simulink model "part2"  (R2018b)
settings: Solver=VariableStepAuto  StartTime=0.0  StopTime=35  FixedStep=0.01  MaxStep=0.01  RelTol=1e-3
undefined symbols (not defined in the file or in its folder): D, DiscIntNeverNeededParam
libraries: simulink x8, Solver_SF x1, dsparch4 x1
(part 2 of 2)

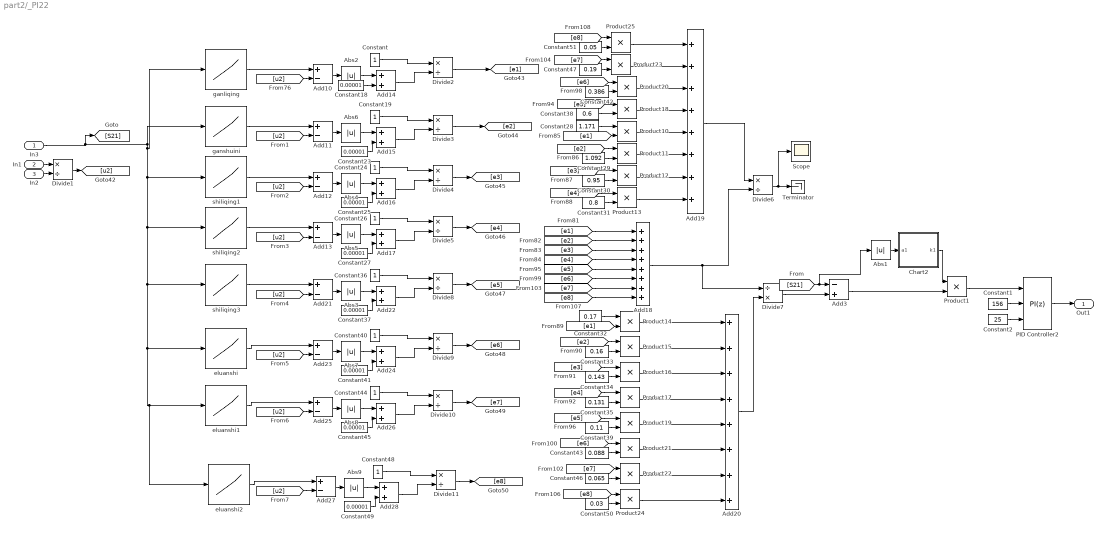
== system part2/_PI22 ==
  In3 : Inport
  In1 : Inport  Port=2
  In2 : Inport  Port=3
  Abs{1..9} (9 alike) : Abs
  Add{10..13,21,23,25,27} (8 alike) : Sum  Inputs=+-
  Add{14..17,22,24,26,28} (8 alike) : Sum
  Add18 : Sum  Inputs=++++++++
  Add19 : Sum  Inputs=++++++++
  Add20 : Sum  Inputs=++++++++
  Add3 : Sum  Inputs=-+
  Chart2 : Stateflow chart  TreatAsAtomicUnit=on
  Constant{,19,24,26,36,40,44,48} (8 alike) : Constant
  Constant1 : Constant  Value=156
  Constant{18,23,25,27,37,41,45,49} (8 alike) : Constant  Value=0.00001
  Constant2 : Constant  Value=25
  Constant28 : Constant  Value=1.171
  Constant29 : Constant  Value=1.092
  Constant30 : Constant  Value=0.95
  Constant31 : Constant  Value=0.8
  Constant32 : Constant  Value=0.17
  Constant33 : Constant  Value=0.16
  Constant34 : Constant  Value=0.143
  Constant35 : Constant  Value=0.131
  Constant38 : Constant  Value=0.6
  Constant39 : Constant  Value=0.11
  Constant42 : Constant  Value=0.386
  Constant43 : Constant  Value=0.088
  Constant46 : Constant  Value=0.065
  Constant47 : Constant  Value=0.19
  Constant50 : Constant  Value=0.03
  Constant51 : Constant  Value=0.05
  Divide{1..6,8..11} (10 alike) : Product  Inputs=*/
  Divide7 : Product  Inputs=/*
  PID Controller2 : simulink/Continuous/PID Controller  Controller=PI  Form=Parallel  TimeDomain=Discrete-time  SampleTime=0.01  IntegratorMethod=Forward Euler  FilterMethod=Forward Euler  ControllerParametersSource=external  P=156  I=25  D=D  UseFilter=on  N=100  TunerSelectOption=Transfer Function Based (PID Tuner App)  InitialConditionSource=internal  InitialConditionForIntegrator=0  InitialConditionForFilter=0  DifferentiatorICPrevScaledInput=0  ExternalReset=none  TrackingMode=off  Kt=1  LimitOutput=on  UpperSaturationLimit=inf  LowerSaturationLimit=-inf  LinearizeAsGain=on  AntiWindupMode=clamping  Kb=1  POutMin=[]  POutMax=[]  IOutMin=[]  IOutMax=[]  DOutMin=[]  DOutMax=[]  NOutMin=[]  NOutMax=[]  SumOutMin=[]  SumOutMax=[]  SaturationOutMin=[]  SaturationOutMax=[]  PParamMin=[]  PParamMax=[]  IParamMin=[]  IParamMax=[]  DParamMin=[]  DParamMax=[]  NParamMin=[]  NParamMax=[]  KbParamMin=[]  KbParamMax=[]  KtParamMin=[]  KtParamMax=[]  KbOutMin=[]  KbOutMax=[]  KtOutMin=[]  KtOutMax=[]  IntegratorOutMin=[]  IntegratorOutMax=[]  FilterOutMin=[]  FilterOutMax=[]  SumI1OutMin=[]  SumI1OutMax=[]  SumI2OutMin=[]  SumI2OutMax=[]  SumI3OutMin=[]  SumI3OutMax=[]  SumI4OutMin=[]  SumI4OutMax=[]  SumDOutMin=[]  SumDOutMax=[]  DifferentiatorOutMin=[]  DifferentiatorOutMax=[]  FilterDiffOutCoefMin=[]  FilterDiffOutCoefMax=[]  ReciprocalOutMin=[]  ReciprocalOutMax=[]  SumDenOutMin=[]  SumDenOutMax=[]  SumNumOutMin=[]  SumNumOutMax=[]  DivideOutMin=[]  DivideOutMax=[]  IntegratorContinuousStateAttributes=''  IntegratorStateMustResolveToSignalObject=off  IntegratorRTWStateStorageClass=Auto  FilterContinuousStateAttributes=''  FilterStateMustResolveToSignalObject=off  FilterRTWStateStorageClass=Auto  ParallelPVariant=ExternalParameters  IdealPVariant=Disabled  IVariant=ExternalParameters  DVariant=Disabled  IntegratorVariant=Discrete  SatVariant=Enabled  AWVariant=DiscClampingParallel  PCopyVariant=Disabled  TRVariant=Disabled  FdbkBlocksVariant=Forward  IdealPFdbkVariant=Disabled  SatFdbkVariant=Disabled  DerivativeFilterVariant=Disabled  NVariant=Disabled  NCopyVariant=Disabled_SignalSpec  FilterICVariant=Disabled  IntegratorICVariant=InternalICs  ExternalResetVariant=Disabled  TRSumVariant=Passthrough  SumFdbkVariant=Disabled  SumVariant=Sum_PI
  Product{1,10..25} (17 alike) : Product
  Scope : Scope
  Terminator : Terminator
  eluanshi : Lookup_n-D  NumberOfTableDimensions=1  BreakpointsForDimension1=[0.00591,0.009,0.01212,0.01856,0.0196,0.02707,0.03557,0.04385,0.05236,0.06524,0.1011,0.13927,0.18595,0.21975,0.26849,0.32574,0.38507,0.44646,0.51635,0.58188,0.63914,0.70697,0.78123,0.86792,0.92103,0.97184,0.993]  Table=[0.04929,0.12757,0.19671,0.25086,0.2838,0.31087,0.34088,0.36501,0.38001,0.38915,0.38915,0.38621,0.38295,0.37414,0.37121,0.36208,0.35588,0.34707,0.33794,0.335,0.32587,0.31707,0.31087,0.2988,0.29293,0.28673,0.2838]  InternalRulePriority=Speed  RndMeth=Simplest  InputSameDT=on
  eluanshi1 : Lookup_n-D  NumberOfTableDimensions=1  BreakpointsForDimension1=|  Table=|  InternalRulePriority=Speed  RndMeth=Simplest  InputSameDT=on
      BreakpointsForDimension1=|
      | [0.00154
      | 0.00798
      | 0.01649
      | 0.0227
      | 0.03121
      | 0.04178
      | 0.05673
      | 0.12433
      | 0.19216
      | 0.26642
      | 0.36598
      | 0.4952
      | 0.61591
      | 0.79388
      | 0.91873
      | 1.00357]
      Table=|
      | [0.04636
      | 0.11257
      | 0.14257
      | 0.17551
      | 0.18465
      | 0.19052
      | 0.19052
      | 0.18758
      | 0.18465
      | 0.17551
      | 0.17258
      | 0.16051
      | 0.15758
      | 0.14551
      | 0.13638
      | 0.1305]
  eluanshi2 : Lookup_n-D  NumberOfTableDimensions=1  BreakpointsForDimension1=|  Table=|  InternalRulePriority=Speed  RndMeth=Simplest  InputSameDT=on
      BreakpointsForDimension1=|
      | [0.00361
      | 0.00798
      | 0.01212
      | 0.01419
      | 0.01856
      | 0.0227
      | 0.02707
      | 0.02914
      | 0.04178
      | 0.09903
      | 0.15836
      | 0.26435
      | 0.37012
      | 0.49934
      | 0.60327
      | 0.69225
      | 0.78537
      | 0.86792
      | 0.94425
      | 1.0015]
      Table=|
      | [0.05549
      | 0.1093
      | 0.13964
      | 0.1517
      | 0.16051
      | 0.16964
      | 0.17845
      | 0.18465
      | 0.19052
      | 0.19052
      | 0.18465
      | 0.17845
      | 0.17258
      | 0.16671
      | 0.15758
      | 0.15464
      | 0.14551
      | 0.14257
      | 0.13638
      | 0.13344]
  ganliqing : Lookup_n-D  NumberOfTableDimensions=1  BreakpointsForDimension1=|  Table=|  InternalRulePriority=Speed  RndMeth=Simplest  InputSameDT=on
      BreakpointsForDimension1=|
      | [0.01498
      | 0.03128
      | 0.05446
      | 0.06846
      | 0.08017
      | 0.09165
      | 0.10335
      | 0.11506
      | 0.12424
      | 0.13595
      | 0.15454
      | 0.16625
      | 0.17772
      | 0.19632
      | 0.22202
      | 0.25691
      | 0.31499
      | 0.38017
      | 0.49196
      | 0.59433
      | 0.70129
      | 0.80367
      | 0.86885
      | 0.95493
      | 0.999]
      Table=|
      | [0.38854
      | 0.66554
      | 0.92268
      | 1.00503
      | 1.04474
      | 1.08738
      | 1.12058
      | 1.13686
      | 1.1502
      | 1.16322
      | 1.1668
      | 1.1668
      | 1.1668
      | 1.16322
      | 1.15346
      | 1.14044
      | 1.11049
      | 1.07762
      | 1.02489
      | 0.9689
      | 0.91617
      | 0.86019
      | 0.82699
      | 0.78435
      | 0.76123]
  ganshuini : Lookup_n-D  NumberOfTableDimensions=1  BreakpointsForDimension1=|  Table=|  InternalRulePriority=Speed  RndMeth=Simplest  InputSameDT=on
      BreakpointsForDimension1=|
      | [0
      | 0.00612
      | 0.01323
      | 0.0185
      | 0.024
      | 0.03293
      | 0.04531
      | 0.05241
      | 0.06295
      | 0.06845
      | 0.07555
      | 0.08266
      | 0.08976
      | 0.0932
      | 0.10213
      | 0.11107
      | 0.12161
      | 0.13055
      | 0.14315
      | 0.15369
      | 0.17156
      | 0.18577
      | 0.19631
      | 0.21419
      | 0.2355
      | 0.25497
      | 0.27468
      | 0.28889
      | 0.30676
      | 0.3173
      | 0.33334
      | 0.35465
      | 0.37252
      | 0.3991
      | 0.41858
      | 0.44539
      | 0.46143
      | 0.48985
      | 0.51299
      | 0.53613
      | 0.55194
      | 0.56798
      | 0.59823
      | 0.6161
      | 0.64085
      | 0.66926
      | 0.69424
      | 0.69791
      | 0.71211
      | 0.75107
      | 0.79209
      | 0.81706
      | 0.85075
      | 0.89887
      | 0.93599
      | 0.98411
      | 0.99832]
      Table=|
      | [0.0357
      | 0.13134
      | 0.30251
      | 0.41079
      | 0.52393
      | 0.63999
      | 0.78847
      | 0.84617
      | 0.90679
      | 0.9444
      | 0.97228
      | 0.99238
      | 1.01248
      | 1.02512
      | 1.04263
      | 1.05787
      | 1.06532
      | 1.07537
      | 1.07797
      | 1.08056
      | 1.08056
      | 1.07797
      | 1.07537
      | 1.06792
      | 1.05527
      | 1.05009
      | 1.04004
      | 1.03258
      | 1.02512
      | 1.01994
      | 1.00989
      | 0.99724
      | 0.98979
      | 0.97455
      | 0.9645
      | 0.94959
      | 0.94181
      | 0.92949
      | 0.91425
      | 0.90161
      | 0.89156
      | 0.8841
      | 0.86886
      | 0.86141
      | 0.84876
      | 0.82867
      | 0.81602
      | 0.81343
      | 0.80857
      | 0.78587
      | 0.76318
      | 0.75313
      | 0.73562
      | 0.70547
      | 0.69024
      | 0.66268
      | 0.6549]
  shiliqing1 : Lookup_n-D  NumberOfTableDimensions=1  BreakpointsForDimension1=|  Table=|  InternalRulePriority=Speed  RndMeth=Simplest  InputSameDT=on
      BreakpointsForDimension1=|
      | [0.00269
      | 0.00429
      | 0.01139
      | 0.01689
      | 0.02033
      | 0.0256
      | 0.0311
      | 0.04004
      | 0.04874
      | 0.06135
      | 0.07372
      | 0.08609
      | 0.0987
      | 0.11451
      | 0.13948
      | 0.1734
      | 0.20342
      | 0.23023
      | 0.24787
      | 0.26391
      | 0.28522
      | 0.30676
      | 0.3173
      | 0.35465
      | 0.39383
      | 0.42935
      | 0.47564
      | 0.51826
      | 0.55905
      | 0.59113
      | 0.63925
      | 0.68003
      | 0.72266
      | 0.7529
      | 0.79552
      | 0.84548
      | 0.89153
      | 0.92545
      | 0.99488]
      Table=|
      | [0.04835
      | 0.16927
      | 0.24707
      | 0.3278
      | 0.39328
      | 0.54662
      | 0.63221
      | 0.70547
      | 0.76059
      | 0.82607
      | 0.87405
      | 0.89901
      | 0.9243
      | 0.93694
      | 0.93954
      | 0.93694
      | 0.92689
      | 0.92171
      | 0.90906
      | 0.9042
      | 0.89415
      | 0.8841
      | 0.87665
      | 0.864
      | 0.84876
      | 0.82867
      | 0.81116
      | 0.79592
      | 0.77323
      | 0.75832
      | 0.74049
      | 0.72298
      | 0.70029
      | 0.69024
      | 0.67014
      | 0.64744
      | 0.62994
      | 0.6147
      | 0.58196]
  shiliqing2 : Lookup_n-D  NumberOfTableDimensions=1  BreakpointsForDimension1=|  Table=|  InternalRulePriority=Speed  RndMeth=Simplest  InputSameDT=on
      BreakpointsForDimension1=|
      | [8.52288E-4
      | 0.00429
      | 0.00612
      | 0.00796
      | 0.01139
      | 0.01506
      | 0.01689
      | 0.0185
      | 0.02033
      | 0.02216
      | 0.0256
      | 0.02927
      | 0.03454
      | 0.0382
      | 0.04164
      | 0.04714
      | 0.05058
      | 0.05768
      | 0.06478
      | 0.07189
      | 0.08082
      | 0.08793
      | 0.0932
      | 0.0987
      | 0.1058
      | 0.1129
      | 0.12528
      | 0.14315
      | 0.1876
      | 0.21052
      | 0.23023
      | 0.25337
      | 0.29072
      | 0.33678
      | 0.40437
      | 0.48435
      | 0.55561
      | 0.6035
      | 0.70662
      | 0.76894
      | 0.84364
      | 0.92018
      | 1.00015]
      Table=|
      | [0.04575
      | 0.09859
      | 0.14139
      | 0.19423
      | 0.24221
      | 0.285
      | 0.33525
      | 0.37059
      | 0.40074
      | 0.43348
      | 0.46622
      | 0.53171
      | 0.56672
      | 0.59201
      | 0.62475
      | 0.65231
      | 0.675
      | 0.71034
      | 0.73789
      | 0.75313
      | 0.77064
      | 0.77842
      | 0.78328
      | 0.78847
      | 0.79592
      | 0.79852
      | 0.79852
      | 0.79333
      | 0.78587
      | 0.77842
      | 0.77064
      | 0.76577
      | 0.75313
      | 0.73562
      | 0.71293
      | 0.68505
      | 0.66009
      | 0.64485
      | 0.6147
      | 0.58715
      | 0.56186
      | 0.53657
      | 0.50902]
  shiliqing3 : Lookup_n-D  NumberOfTableDimensions=1  BreakpointsForDimension1=|  Table=|  InternalRulePriority=Speed  RndMeth=Simplest  InputSameDT=on
      BreakpointsForDimension1=|
      | [0.0
      | 0.00154
      | 0.00798
      | 0.01212
      | 0.01419
      | 0.01856
      | 0.02477
      | 0.02914
      | 0.03764
      | 0.04615
      | 0.05236
      | 0.05673
      | 0.06087
      | 0.06937
      | 0.07788
      | 0.08846
      | 0.10317
      | 0.11812
      | 0.1372
      | 0.16893
      | 0.20503
      | 0.24941
      | 0.29171
      | 0.32988
      | 0.37012
      | 0.41243
      | 0.45496
      | 0.49083
      | 0.529
      | 0.57775
      | 0.62856
      | 0.68167
      | 0.73249
      | 0.77686
      | 0.82975
      | 0.90608
      | 0.94839
      | 1]
      Table=|
      | [0.0
      | 0.09756
      | 0.14551
      | 0.20878
      | 0.25379
      | 0.32
      | 0.35588
      | 0.39208
      | 0.44329
      | 0.47917
      | 0.50624
      | 0.5245
      | 0.5395
      | 0.55451
      | 0.57245
      | 0.58158
      | 0.59071
      | 0.59952
      | 0.59658
      | 0.59365
      | 0.58745
      | 0.57864
      | 0.57245
      | 0.56364
      | 0.55451
      | 0.54831
      | 0.5395
      | 0.53331
      | 0.5245
      | 0.51537
      | 0.5033
      | 0.49417
      | 0.48536
      | 0.47623
      | 0.46416
      | 0.44916
      | 0.44329
      | 0.43122]
  Out1 : Outport
  wires:
  Divide1/1 -> [u2]
  In2/1 -> Divide1/2
  In1/1 -> Divide1/1
  [u2] -> Add11/2
  Add12/1 -> Abs4/1
  [e1] -> Product14/2
  [e3] -> Product12/1
  Constant18/1 -> Add14/2
  ganliqing/1 -> Add10/1
  Constant/1 -> Divide2/1
  eluanshi2/1 -> Add27/1
  [e5] -> Product19/1
  Divide11/1 -> [e8]
  Product22/1 -> Add20/7
  Add10/1 -> Abs2/1
  shiliqing1/1 -> Add12/1
  eluanshi1/1 -> Add25/1
  Constant48/1 -> Divide11/1
  Constant28/1 -> Product10/1
  Product20/1 -> Add19/3
  [u2] -> Add25/2
  Product21/1 -> Add20/6
  Constant50/1 -> Product24/2
  [e8] -> Product24/1
  [e8] -> Product25/1
  Add21/1 -> Abs3/1
  [e7] -> Product23/1
  Product19/1 -> Add20/5
  [e7] -> Add18/7
  Divide4/1 -> [e3]
  Add26/1 -> Divide10/2
  Add28/1 -> Divide11/2
  Add25/1 -> Abs8/1
  Add27/1 -> Abs9/1
  Constant36/1 -> Divide8/1
  Product16/1 -> Add20/3
  [e1] -> Product10/2
  [u2] -> Add27/2
  Product23/1 -> Add19/2
  Constant51/1 -> Product25/2
  [e3] -> Product16/1
  [u2] -> Add23/2
  Constant47/1 -> Product23/2
  Add24/1 -> Divide9/2
  Add18/1 -> Divide7/1, Divide6/2
  Divide10/1 -> [e7]
  [e4] -> Product13/1
  Constant32/1 -> Product14/1
  [e6] -> Add18/6
  Constant39/1 -> Product19/2
  Abs7/1 -> Add24/1
  Product14/1 -> Add20/1
  Product11/1 -> Add19/6
  Add22/1 -> Divide8/2
  Constant43/1 -> Product21/2
  Constant44/1 -> Divide10/1
  Constant38/1 -> Product18/2
  eluanshi/1 -> Add23/1
  Constant45/1 -> Add26/2
  [e2] -> Product15/1
  Constant41/1 -> Add24/2
  Add20/1 -> Divide7/2
  Constant37/1 -> Add22/2
  In3/1 -> [S21], eluanshi2/1, eluanshi1/1, eluanshi/1, shiliqing3/1, shiliqing2/1, shiliqing1/1, ganliqing/1, ganshuini/1
  [u2] -> Add12/2
  Constant33/1 -> Product15/2
  Constant35/1 -> Product17/2
  Divide3/1 -> [e2]
  Constant46/1 -> Product22/2
  [e4] -> Product17/1
  Add19/1 -> Divide6/1
  Divide9/1 -> [e6]
  Constant30/1 -> Product12/2
  [e5] -> Add18/5
  Add23/1 -> Abs7/1
  Constant23/1 -> Add15/2
  Constant27/1 -> Add17/2
  [e5] -> Product18/1
  [e1] -> Add18/1
  Constant26/1 -> Divide5/1
  Product12/1 -> Add19/7
  Constant34/1 -> Product16/2
  Product18/1 -> Add19/4
  ganshuini/1 -> Add11/1
  Product15/1 -> Add20/2
  shiliqing3/1 -> Add21/1
  Constant31/1 -> Product13/2
  Constant24/1 -> Divide4/1
  Constant25/1 -> Add16/2
  [u2] -> Add21/2
  Add17/1 -> Divide5/2
  Abs5/1 -> Add17/1
  Abs6/1 -> Add15/1
  Abs2/1 -> Add14/1
  [e6] -> Product21/1
  [e2] -> Add18/2
  [u2] -> Add13/2
  Add15/1 -> Divide3/2
  Divide5/1 -> [e4]
  Product10/1 -> Add19/5
  Abs9/1 -> Add28/1
  Constant19/1 -> Divide3/1
  Constant40/1 -> Divide9/1
  [e7] -> Product22/1
  Abs4/1 -> Add16/1
  Abs8/1 -> Add26/1
  [e2] -> Product11/1
  Add16/1 -> Divide4/2
  [e4] -> Add18/4
  Divide8/1 -> [e5]
  [e3] -> Add18/3
  Constant29/1 -> Product11/2
  Abs3/1 -> Add22/1
  Add11/1 -> Abs6/1
  [e6] -> Product20/1
  shiliqing2/1 -> Add13/1
  [u2] -> Add10/2
  Constant42/1 -> Product20/2
  Add14/1 -> Divide2/2
  Product13/1 -> Add19/8
  Add13/1 -> Abs5/1
  Product17/1 -> Add20/4
  Divide2/1 -> [e1]
  Constant49/1 -> Add28/2
  Add3/1 -> Product1/2
  Abs1/1 -> Chart2/1(a1)
  Chart2/1(k1) -> Product1/1
  Divide6/1 -> Scope/1, Terminator/1
  Product1/1 -> PID Controller2/1
  Constant1/1 -> PID Controller2/2
  Constant2/1 -> PID Controller2/3
  Divide7/1 -> Add3/2
  [S21] -> Abs1/1, Add3/1
  PID Controller2/1 -> Out1/1
  Product25/1 -> Add19/1
  [e8] -> Add18/8
  Product24/1 -> Add20/8

== stateflow chart part2/PID/Chart2 ==
  (default) -> (junction 1)
  (junction 1) -> (junction 5) [order 1] : [a1>1
      | ]
  (junction 1) -> (junction 9) [order 2]
  (junction 5) -> (junction 7) : {k1=1;}
  (junction 7) -> (junction 9)
  (junction 9) -> (junction 12)
  (junction 12) -> (junction 14) [order 1] : [a1<=1]
  (junction 12) -> (junction 19) [order 2]
  (junction 14) -> (junction 16) : {k1=0;}
  (junction 16) -> (junction 19)
  data: a1 input; k1 output

== stateflow chart part2/PID/Chart1 ==
  (default) -> (junction 1)
  (junction 1) -> (junction 5) [order 1] : [a1>1
      | ]
  (junction 1) -> (junction 9) [order 2]
  (junction 5) -> (junction 7) : {k1=1;}
  (junction 7) -> (junction 9)
  (junction 9) -> (junction 12)
  (junction 12) -> (junction 14) [order 1] : [a1<=1]
  (junction 12) -> (junction 19) [order 2]
  (junction 14) -> (junction 16) : {k1=0;}
  (junction 16) -> (junction 19)
  data: a1 input; k1 output

== stateflow chart part2/_PI21/Chart2 ==
  (default) -> (junction 1)
  (junction 1) -> (junction 5) [order 1] : [a1>=0.1
      | ]
  (junction 5) -> (junction 37) : {k = k + 1;}
  (junction 1) -> (junction 37) [order 2]
  (junction 37) -> (junction 40)
  (junction 40) -> (junction 39) [order 1] : [a1<0.1
      | ]
  (junction 40) -> (junction 42) [order 2]
  (junction 39) -> (junction 41) : {k=0;k1=0;}
  (junction 41) -> (junction 42)
  (junction 42) -> (junction 9)
  (junction 9) -> (junction 32) [order 1] : [k>=3]
  (junction 32) -> (junction 30) : {k1=1;}
  (junction 9) -> (junction 30) [order 2]
  data: a1 input; k1 output; a local; k local =0

== stateflow chart part2/_PI22/Chart2 ==
  (default) -> (junction 1)
  (junction 1) -> (junction 5) [order 1] : [a1>=0.1
      | ]
  (junction 5) -> (junction 37) : {k = k + 1;}
  (junction 1) -> (junction 37) [order 2]
  (junction 37) -> (junction 40)
  (junction 40) -> (junction 39) [order 1] : [a1<0.1
      | ]
  (junction 40) -> (junction 42) [order 2]
  (junction 39) -> (junction 41) : {k=0;k1=0;}
  (junction 41) -> (junction 42)
  (junction 42) -> (junction 9)
  (junction 9) -> (junction 32) [order 1] : [k>=3]
  (junction 32) -> (junction 30) : {k1=1;}
  (junction 9) -> (junction 30) [order 2]
  data: a1 input; k1 output; a local; k local =0

== matlab function part2/MATLAB Function ==
  data: vx input; delta input; u input; wz_exp output; beta_exp output
function [wz_exp,beta_exp] = Two_dof(vx,delta,u)
m=345.5; %整车质量kg
Lf=1.56*0.55; %质心距离前轴的距离m 1.27
Lr=1.56*0.45; %质心距离后轴的距离m
L=Lf+Lr; %轴距m
Iz=540; %整车z轴转动惯量kg*m^2
k1=-151;%两前轮侧偏刚度之和 N/rad
k2=-147;%两后轮侧偏刚度之和 N/rad
c1=k1*L/(m*Lr); %侧偏系数 1/rad
c2=k2*L/(m*Lf);
K=-(1/c1-1/c2)/L;


wz_exp = (min(abs(vx*delta/(L*(1+K*vx^2))),abs(0.85*u*9.8/vx)))*sign(delta);
beta_exp= (min(abs(((Lr/L+m*Lf*vx^2/(L^2*k1))/(1+K*vx^2))*delta),abs(u*9.8*(Lr/vx^2+m*Lf/k2/L))))*sign(((Lr/L+m*Lf*vx^2/(L^2*k1))/(1+K*vx^2))*delta);
